simulink model "fuzzy_P"  (R2022b)
settings: Solver=VariableStepAuto  StartTime=0.0  StopTime=50  RelTol=1e-3
libraries: fuzblock x1
settings Model: Creator=sophy  LastModifiedBy=sophy

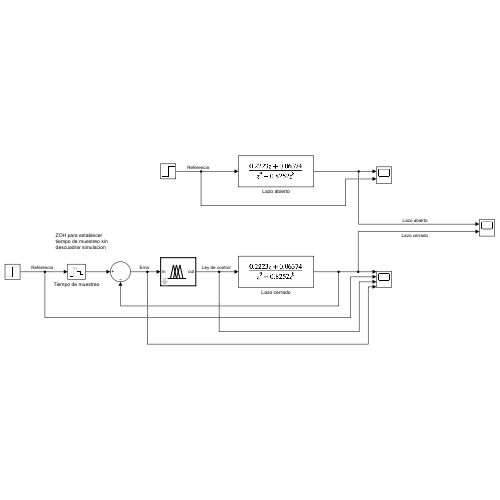
[thumbnail: Simulink's stored preview of the top-level diagram]
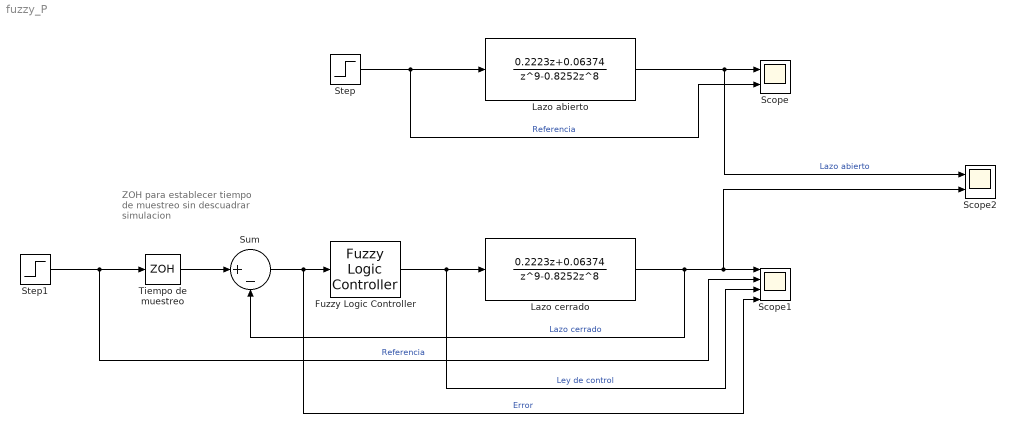
== system fuzzy_P ==
  note: ZOH para establecer tiempo de muestreo sin descuadrar simulacion
  Fuzzy Logic Controller : fuzblock/Fuzzy Logic  Controller  FIS=mamdanitype1  OutputSampleNumber=101  DataType=double  FuzzifiedInputs=off  RuleFiringStrengths=off  RuleOutputs=off  AggregatedOutputs=off  SimulateUsing=Interpreted execution  OutOfRangeInputValueMessage=warning  NoRuleFiredMessage=warning  EmptyOutputFuzzySetMessage=warning
  Lazo abierto : DiscreteTransferFcn  Numerator=[0.2223 0.06374]  Denominator=[1 -0.8252 0 0 0 0 0 0 0 0]
  Lazo cerrado : DiscreteTransferFcn  Numerator=[0.2223 0.06374]  Denominator=[1 -0.8252 0 0 0 0 0 0 0 0]
  Scope : Scope  NumInputPorts=2
  Scope1 : Scope  NumInputPorts=4
  Scope2 : Scope  NumInputPorts=2
  Step : Step  After=50  SampleTime=0
  Step1 : Step  After=50  SampleTime=0
  Sum : Sum  Inputs=|+-
  Tiempo de muestreo : ZeroOrderHold  SampleTime=0.1412
  wires:
  Step/1 -> Scope/2, Lazo abierto/1  "Referencia"
  Lazo abierto/1 -> Scope2/1, Scope/1  "Lazo abierto"
  Fuzzy Logic Controller/1 -> Scope1/3, Lazo cerrado/1  "Ley de control"
  Sum/1 -> Scope1/4, Fuzzy Logic Controller/1  "Error"
  Step1/1 -> Tiempo de muestreo/1, Scope1/2  "Referencia"
  Lazo cerrado/1 -> Scope2/2, Scope1/1, Sum/2  "Lazo cerrado"
  Tiempo de muestreo/1 -> Sum/1
